simulink model "M12_MIMO_flexBitLoad_SVD"  (R2021a)
settings: Solver=FixedStepDiscrete  StartTime=0.0  StopTime=inf  RelTol=1e-3  EnableMultiTasking=on
undefined symbols (not defined in the file): B1, B2, BER, delay1, delay2, gcbh, L, magnitude, pl, pl1, pl2, rcfiltgaincompat, S, sigM1_g, sigM2_g, sigma, System, Tbit5_0, Tsk
libraries: simulink x8, dspstat3 x8, commfilt2 x4, commutil2 x2, commrandsrc3 x2, commdigbbndam3 x2, commsink2 x2, GeneralASKLib x2, NoiseLib_2021 x1, dspsrcs4 x1
settings Model: Creator=Praktikum  LastModifiedBy=st181028
settings SolverCC: AlgebraicLoopSolver=TrustRegion
settings DataIOCC: LimitDataPoints=on  SaveFormat=Array
settings OptimizationCC: ExpressionDepthLimit=2147483647  InitFltsAndDblsToZero=on  LifeSpan=inf
settings DebuggingCC: SaveWithDisabledLinksMsg=none  SaveWithParameterizedLinksMsg=none  SignalResolutionControl=TryResolveAllWithWarning  SolverPrmCheckMsg=warning  MultiTaskDSMMsg=warning  MultiTaskCondExecSysMsg=none  StateNameClashWarn=warning  StrictBusMsg=ErrorOnBusTreatedAsVector  SFUnexpectedBacktrackingDiag=warning  SFNoUnconditionalDefaultTransitionDiag=warning  SFMachineParentedDataDiag=warning  ArithmeticOperatorsInVariantConditions=warning
settings HardwareCC: ProdBitPerPointer=32  ProdBitPerSizeT=32  ProdBitPerPtrDiffT=32  ProdLargestAtomicFloat=None  ProdIntDivRoundTo=Undefined  ProdEndianess=Unspecified  ProdWordSize=32  ProdHWDeviceType=32-bit Generic
settings ModelReferenceCC: PropagateSignalLabelsOutOfModel=off
settings SFSimCC: SimUseLocalCustomCode=off  SimParseCustomCode=off  CustomCodeUndefinedFunction=UseInterfaceOnly
settings RTWCC: RTWUseLocalCustomCode=off
settings CodeAppCC: StateflowObjectComments=on
settings GRTTargetCC: TargetFcnLib=ansi_tfl_tmw.mat  TargetLangStandard=C89/C90 (ANSI)  CombineOutputUpdateFcns=off  GRTInterface=on
settings ConfigComp: CovMetricSettings=dw  CovSaveCumulativeToWorkspaceVar=on  CovSaveSingleToWorkspaceVar=on  CovExternalEMLEnable=off  CovSFcnEnable=off

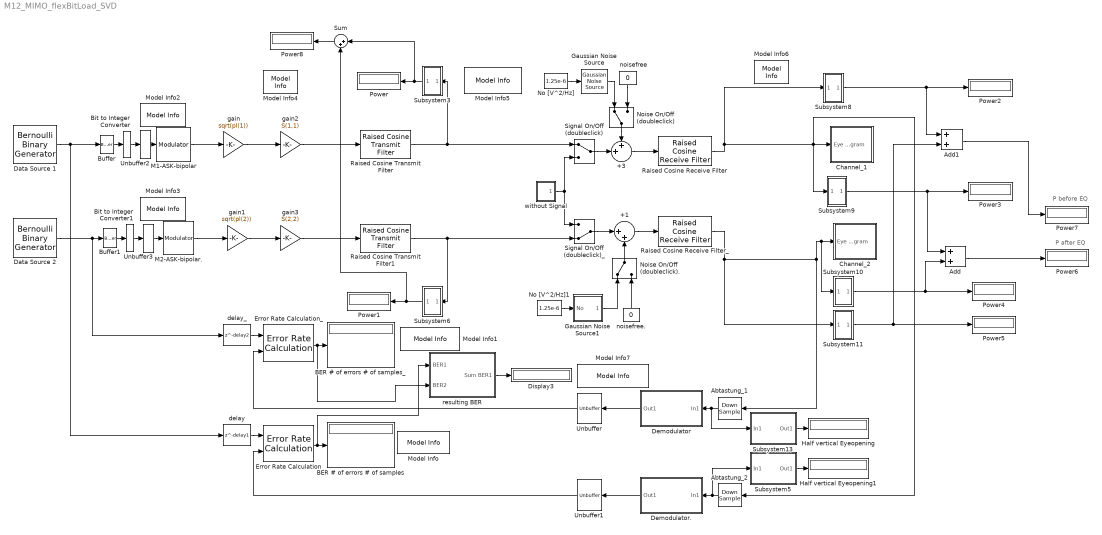
== system M12_MIMO_flexBitLoad_SVD ==
  note: P after EQ
  note: P before EQ
   Power{,1..8} (9 alike) : Display
  +1 : Sum  Inputs=|++  SampleTime=Tbit5_0/16
  +3 : Sum  Inputs=++|  SampleTime=Tbit5_0/16
  Abtastung_1 : DownSample  N=16  RateOptions=Allow multirate processing
  Abtastung_2 : DownSample  N=16  RateOptions=Allow multirate processing
  Add : Sum
  Add1 : Sum
  BER # of errors # of samples : Display
      settings: Format=short_e  Decimation=2
  BER # of errors # of samples_ : Display
      settings: Format=short_e  Decimation=2
  Bit to Integer Converter : commutil2/Bit to Integer Converter  nbits=B1  bitOrder=MSB first  signedOutputValues=Unsigned  outDtype=Inherit via internal rule  outDtypeSigned=Inherit via internal rule
  Bit to Integer Converter1 : commutil2/Bit to Integer Converter  nbits=B2  bitOrder=MSB first  signedOutputValues=Unsigned  outDtype=Inherit via internal rule  outDtypeSigned=Inherit via internal rule
  Buffer : Buffer  N=B1
  Buffer1 : Buffer  N=B2
  Channel_1 : Subsystem
  Channel_2 : Subsystem
  Data Source 1 : commrandsrc3/Bernoulli Binary Generator  ProbabilityOfZero=0.5  SeedSource=Parameter  Seed=61  SampleTime=Tbit5_0/B1  SamplesPerFrame=1  OutputDataType=double  SimulateUsing=Interpreted execution
  Data Source 2 : commrandsrc3/Bernoulli Binary Generator  ProbabilityOfZero=0.5  SeedSource=Parameter  Seed=51  SampleTime=Tbit5_0/B2  SamplesPerFrame=1  OutputDataType=double  SimulateUsing=Interpreted execution
  Demodulator : Subsystem  AncestorBlock=GeneralASKLib/Demodulator
      mask Display:
      | plot(0,0,100,100,[20+1.5*[[0:.8:10] [10:1.6:20] [20:.8:30]] 65 65 65 65+10*[0 1 1 2 2 3]],[85+10*[sin([0:.8:10]*pi*2/5) sin([10:1.6:20]*pi/5) sin([20:.8:30]*pi*2/5)] 85 99 75 85+8*[1 1 -1 -1 1 1]]);
      | disp('\nGeneral\nASK-Demodulator')
  Demodulator. : Subsystem  AncestorBlock=GeneralASKLib/Demodulator
      mask Display:
      | plot(0,0,100,100,[20+1.5*[[0:.8:10] [10:1.6:20] [20:.8:30]] 65 65 65 65+10*[0 1 1 2 2 3]],[85+10*[sin([0:.8:10]*pi*2/5) sin([10:1.6:20]*pi/5) sin([20:.8:30]*pi*2/5)] 85 99 75 85+8*[1 1 -1 -1 1 1]]);
      | disp('\nGeneral\nASK-Demodulator')
  Display3 : Display
      settings: Format=short_e
  Error Rate Calculation : commsink2/Error Rate Calculation  N=0  st_delay=100  cp_mode=Entire frame  subframe=1  PMode=Port  WsName=ErrorVec  RsMode2=off  stop=off  numErr=100  maxBits=1e6
  Error Rate Calculation_ : commsink2/Error Rate Calculation  N=0  st_delay=100  cp_mode=Entire frame  subframe=1  PMode=Port  WsName=ErrorVec  RsMode2=off  stop=off  numErr=100  maxBits=1e6
  Gaussian Noise Source : NoiseLib_2021/Gaussian Noise Source  SystemSampleTime=-1  VariantActivationTime=update diagram  Latency=0  AutoFrameSizeCalculation=off
  Gaussian Noise Source1 : Subsystem  AncestorBlock=NoiseLib_2021/Gaussian Noise Source
      mask Display:
      | plot(0,0,100,100,[95 5 10 10 10 (100-15)*[0:1/30:1]+10],[75 75 75 70 95 70    58 76 77 63 86 86 74 78 76 73 82 69 96 73 76 85 75 74 66 77 61 82 91 68    83 87 59 60 80 71]);
      | disp('\n\nGaussian')
      | port_label('input',1,'No')
      | port_label('output',1,'noise')
  Half vertical Eyeopening : Display
  Half vertical Eyeopening1 : Display
  M1-ASK-bipolar : GeneralASKLib/Modulator  SystemSampleTime=-1  VariantActivationTime=update diagram  Latency=0  AutoFrameSizeCalculation=off
      link override General ASK Modulator Baseband: SigCon=[sigM1_g]
  M2-ASK-bipolar. : GeneralASKLib/Modulator  SystemSampleTime=-1  VariantActivationTime=update diagram  Latency=0  AutoFrameSizeCalculation=off
      link override General ASK Modulator Baseband: SigCon=[sigM2_g]
  Model Info : simulink/Model-Wide Utilities/Model Info  Frame=off  DisplayStringWithTags=Channel_1  HorizontalTextAlignment=Center  LeftAlignmentValue=0.5
  Model Info1 : simulink/Model-Wide Utilities/Model Info  Frame=off  DisplayStringWithTags=Channel_2  HorizontalTextAlignment=Center  LeftAlignmentValue=0.5
  Model Info2 : simulink/Model-Wide Utilities/Model Info  Frame=off  DisplayStringWithTags=Channel1  HorizontalTextAlignment=Center  LeftAlignmentValue=0.5
  Model Info3 : simulink/Model-Wide Utilities/Model Info  Frame=off  DisplayStringWithTags=Channel2  HorizontalTextAlignment=Center  LeftAlignmentValue=0.5
  Model Info4 : simulink/Model-Wide Utilities/Model Info  Frame=off  DisplayStringWithTags=pre  HorizontalTextAlignment=Center  LeftAlignmentValue=0.5
  Model Info5 : simulink/Model-Wide Utilities/Model Info  Frame=off  DisplayStringWithTags=H  HorizontalTextAlignment=Center  LeftAlignmentValue=0.5
  Model Info6 : simulink/Model-Wide Utilities/Model Info  Frame=off  DisplayStringWithTags=pst  HorizontalTextAlignment=Center  LeftAlignmentValue=0.5
  Model Info7 : simulink/Model-Wide Utilities/Model Info  Frame=off  DisplayStringWithTags=System-BER  HorizontalTextAlignment=Center  LeftAlignmentValue=0.5
  No [V^2/Hz] : Constant  Value=1.25e-6
  No [V^2/Hz]1 : Constant  Value=1.25e-6
  Noise On/Off (doubleclick) : ManualSwitch
  Noise On/Off (doubleclick). : ManualSwitch
  Raised Cosine Receive Filter : commfilt2/Raised Cosine Receive Filter  filtType=Square root  R=0.5  filtSpan=2*(4)  N=16  downFactor=1  downOffset=0  filterGain=(0.25)*rcfiltgaincompat(gcbh)  RateOptions=Allow multirate processing  framing=Mute  checkCoeff=off  variableName=rcRxFilt  currentFiltSpan=2*(4)  D=4  inputOffset=0  sampMode=Mute  saveAsFlag=0  rateMode=Downsampling  checkGain=User-specified  launchFVT=off  roundingMode=Floor  overflowMode=off  coeffDataTypeStr=Inherit: Same word length as input  coeffMin=[]  coeffMax=[]  coeffLastDataTypeStr=Inherit: Same word length as input  accumDataTypeStr=Inherit: Same as product output  accumLastDataTypeStr=Inherit: Same as product output  outputDataTypeStr=Inherit: Same as accumulator  outputMin=[]  outputMax=[]  outputLastDataTypeStr=Inherit: Same as accumulator
  Raised Cosine Receive Filter_ : commfilt2/Raised Cosine Receive Filter  filtType=Square root  R=0.5  filtSpan=2*(4)  N=16  downFactor=1  downOffset=0  filterGain=(0.25)*rcfiltgaincompat(gcbh)  RateOptions=Allow multirate processing  framing=Mute  checkCoeff=off  variableName=rcRxFilt1  currentFiltSpan=2*(4)  D=4  inputOffset=0  sampMode=Mute  saveAsFlag=0  rateMode=Downsampling  checkGain=User-specified  launchFVT=off  roundingMode=Floor  overflowMode=off  coeffDataTypeStr=Inherit: Same word length as input  coeffMin=[]  coeffMax=[]  coeffLastDataTypeStr=Inherit: Same word length as input  accumDataTypeStr=Inherit: Same as product output  accumLastDataTypeStr=Inherit: Same as product output  outputDataTypeStr=Inherit: Same as accumulator  outputMin=[]  outputMax=[]  outputLastDataTypeStr=Inherit: Same as accumulator
  Raised Cosine Transmit Filter : commfilt2/Raised Cosine Transmit Filter  filtType=Square root  R=0.5  filtSpan=2*(4)  N=16  filterGain=(4/sqrt(2))*rcfiltgaincompat(gcbh)  RateOptions=Allow multirate processing  framing=Mute  checkCoeff=off  variableName=rcTxFilt  checkGain=User-specified  sampMode=Mute  saveAsFlag=0  currentFiltSpan=2*(4)  D=4  launchFVT=off  roundingMode=Floor  overflowMode=off  coeffDataTypeStr=Inherit: Same word length as input  coeffMin=[]  coeffMax=[]  coeffLastDataTypeStr=Inherit: Same word length as input  outputDataTypeStr=Inherit: Same as accumulator  outputMin=[]  outputMax=[]  outputLastDataTypeStr=Inherit: Same as accumulator
  Raised Cosine Transmit Filter1 : commfilt2/Raised Cosine Transmit Filter  filtType=Square root  R=0.5  filtSpan=2*(4)  N=16  filterGain=(4/sqrt(2))*rcfiltgaincompat(gcbh)  RateOptions=Allow multirate processing  framing=Mute  checkCoeff=off  variableName=rcTxFilt1  checkGain=User-specified  sampMode=Mute  saveAsFlag=0  currentFiltSpan=2*(4)  D=4  launchFVT=off  roundingMode=Floor  overflowMode=off  coeffDataTypeStr=Inherit: Same word length as input  coeffMin=[]  coeffMax=[]  coeffLastDataTypeStr=Inherit: Same word length as input  outputDataTypeStr=Inherit: Same as accumulator  outputMin=[]  outputMax=[]  outputLastDataTypeStr=Inherit: Same as accumulator
  Signal On/Off (doubleclick) : ManualSwitch
  Signal On/Off (doubleclick)_ : ManualSwitch  CurrentSetting=0
  Subsystem10 : Subsystem
      mask Display: disp('Power\n Measurement')
  Subsystem11 : Subsystem
      mask Display: disp('Power\n Measurement')
  Subsystem13 : Subsystem
      mask Display:
      | image('eye.bmp','center')
      | disp('\n\n\nEye Opening')
  Subsystem3 : Subsystem
      mask Display: disp('Power\n Measurement')
  Subsystem5 : Subsystem
      mask Display:
      | image('eye.bmp','center')
      | disp('\n\n\nEye Opening')
  Subsystem6 : Subsystem
      mask Display: disp('Power\n Measurement')
  Subsystem8 : Subsystem
      mask Display: disp('Power\n Measurement')
  Subsystem9 : Subsystem
      mask Display: disp('Power\n Measurement')
  Sum : Sum  Inputs=|++
  Unbuffer{,1..3} (4 alike) : Unbuffer
  delay : Delay  DelayLength=delay1  InitialCondition=0  InputProcessing=Columns as channels (frame based)
  delay_ : Delay  DelayLength=delay2  InitialCondition=0  InputProcessing=Columns as channels (frame based)
  gain : Gain  Gain=sqrt(pl(1))
  gain1 : Gain  Gain=sqrt(pl(2))
  gain2 : Gain  Gain=S(1,1)
  gain3 : Gain  Gain=S(2,2)
  noisefree : Constant  Value=0
  noisefree. : Constant  Value=0
  resulting BER : Subsystem
  without Signal : Subsystem
      mask Display: disp('0')
  wires:
  +3/1 -> Raised Cosine Receive Filter/1
  Signal On/Off (doubleclick)/1 -> +3/2
  Error Rate Calculation_/1 -> resulting BER/2(BER2), BER # of errors # of samples_/1
  delay_/1 -> Error Rate Calculation_/1
  Raised Cosine Transmit Filter/1 -> Signal On/Off (doubleclick)/1, Subsystem3/1(In1)
  without Signal/1(Out1) -> Signal On/Off (doubleclick)_/1, Signal On/Off (doubleclick)/2
  Raised Cosine Transmit Filter1/1 -> Signal On/Off (doubleclick)_/2, Subsystem6/1(In1)
  Error Rate Calculation/1 -> resulting BER/1(BER1), BER # of errors # of samples/1
  delay/1 -> Error Rate Calculation/1
  Raised Cosine Receive Filter_/1 -> Subsystem10/1(In1), Channel_2/1(Eye Diagram), Abtastung_1/1, Subsystem11/1(In1)
  Raised Cosine Receive Filter/1 -> Subsystem9/1(In1), Channel_1/1(Eye Diagram), Abtastung_2/1, Subsystem8/1(In1)
  Noise On/Off (doubleclick)/1 -> +3/1
  Abtastung_2/1 -> Subsystem5/1(In1), Demodulator./1(In1)
  Abtastung_1/1 -> Demodulator/1(In1), Subsystem13/1(In1)
  noisefree/1 -> Noise On/Off (doubleclick)/2
  No [V^2/Hz]/1 -> Gaussian Noise Source/1
  Gaussian Noise Source/1 -> Noise On/Off (doubleclick)/1
  Subsystem8/1(Out1) -> Add1/1, " Power2"/1
  Subsystem9/1(Out1) -> Add/1, " Power3"/1
  Subsystem10/1(Out1) -> Add/2, " Power4"/1
  Subsystem11/1(Out1) -> Add1/2, " Power5"/1
  Subsystem13/1(Out1) -> Half vertical Eyeopening/1
  Subsystem5/1(Out1) -> Half vertical Eyeopening1/1
  Subsystem3/1(Out1) -> Sum/1, " Power"/1
  Subsystem6/1(Out1) -> Sum/2, " Power1"/1
  +1/1 -> Raised Cosine Receive Filter_/1
  Signal On/Off (doubleclick)_/1 -> +1/1
  Noise On/Off (doubleclick)./1 -> +1/2
  noisefree./1 -> Noise On/Off (doubleclick)./2
  No [V^2/Hz]1/1 -> Gaussian Noise Source1/1(No)
  Gaussian Noise Source1/1(Noise) -> Noise On/Off (doubleclick)./1
  Unbuffer2/1 -> M1-ASK-bipolar/1
  Buffer/1 -> Bit to Integer Converter/1
  Bit to Integer Converter/1 -> Unbuffer2/1
  Unbuffer3/1 -> M2-ASK-bipolar./1
  Buffer1/1 -> Bit to Integer Converter1/1
  Bit to Integer Converter1/1 -> Unbuffer3/1
  resulting BER/1(Sum BER1) -> Display3/1
  Demodulator/1(Out1) -> Unbuffer/1
  Demodulator./1(Out1) -> Unbuffer1/1
  Unbuffer1/1 -> Error Rate Calculation/2
  Unbuffer/1 -> Error Rate Calculation_/2
  Add/1 -> " Power6"/1
  Add1/1 -> " Power7"/1
  Sum/1 -> " Power8"/1
  M1-ASK-bipolar/1 -> gain/1
  M2-ASK-bipolar./1 -> gain1/1
  Data Source 1/1 -> delay/1, Buffer/1
  Data Source 2/1 -> delay_/1, Buffer1/1
  gain/1 -> gain2/1
  gain2/1 -> Raised Cosine Transmit Filter/1
  gain1/1 -> gain3/1
  gain3/1 -> Raised Cosine Transmit Filter1/1

== system M12_MIMO_flexBitLoad_SVD/Channel_1 ==
  Eye Diagram : Inport
  Discrete-Time Eye Diagram Scope : EyeDiagram  Tag=EyeDiagram
  Realteil : ComplexToRealImag  Output=Real
  wires:
  Eye Diagram/1 -> Realteil/1
  Realteil/1 -> Discrete-Time Eye Diagram Scope/1

== system M12_MIMO_flexBitLoad_SVD/Channel_2 ==
  Eye Diagram : Inport
  Discrete-Time Eye Diagram Scope : EyeDiagram  Tag=EyeDiagram
  Realteil : ComplexToRealImag  Output=Real
  wires:
  Eye Diagram/1 -> Realteil/1
  Realteil/1 -> Discrete-Time Eye Diagram Scope/1

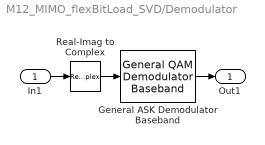
== system M12_MIMO_flexBitLoad_SVD/Demodulator ==
  In1 : Inport
  General ASK Demodulator Baseband : commdigbbndam3/General QAM Demodulator Baseband  SigCon=sigma(2)*sqrt(1/L)*sqrt(pl2)*sigM2_g  OutType=Bit  DecType=Hard decision  VarSource=Dialog  Variance=1  outDtypeBit=Inherit via internal rule  outDtype=Inherit via internal rule  roundingMode=Floor  overflowMode=Wrap  OvFlMode=off  OvFlModeLastStrValue=off  sigConstWordLen=16  sigConstDataTypeStr=Inherit: Same word length as input  sigConstLastDataTypeStr=Inherit: Same word length as input  accum1WordLen=32  accum1FracLen=30  prodInWordLen=32  prodInFracLen=30  prodInDataTypeStr=Inherit: Same as accumulator 1  prodInLastDataTypeStr=Inherit: Same as accumulator 1  prodOutWordLen=32  prodOutFracLen=30  accum2WordLen=32  accum2FracLen=30  accum3WordLen=32  accum3FracLen=30  nsiWordLen=32  nsiFracLen=30  nsiDataTypeStr=Inherit: Same as accumulator 3  nsiLastDataTypeStr=Inherit: Same as accumulator 3  invn0WordLen=16  invn0FracLen=8  invn0DataTypeStr=Inherit: Same word length as input  invn0LastDataTypeStr=Inherit: Same word length as input  outputWordLen=32  outputFracLen=30
      settings: SourceProductBaseCode=CM
  Real-Imag to Complex : RealImagToComplex  Input=Real
  Out1 : Outport
  wires:
  Real-Imag to Complex/1 -> General ASK Demodulator Baseband/1
  General ASK Demodulator Baseband/1 -> Out1/1
  In1/1 -> Real-Imag to Complex/1

== system M12_MIMO_flexBitLoad_SVD/Demodulator. ==
  In1 : Inport
  General ASK Demodulator Baseband : commdigbbndam3/General QAM Demodulator Baseband  SigCon=sigma(1)*sqrt(1/L)*sqrt(pl1)*sigM1_g  OutType=Bit  DecType=Hard decision  VarSource=Dialog  Variance=1  outDtypeBit=Inherit via internal rule  outDtype=Inherit via internal rule  roundingMode=Floor  overflowMode=Wrap  OvFlMode=off  OvFlModeLastStrValue=off  sigConstWordLen=16  sigConstDataTypeStr=Inherit: Same word length as input  sigConstLastDataTypeStr=Inherit: Same word length as input  accum1WordLen=32  accum1FracLen=30  prodInWordLen=32  prodInFracLen=30  prodInDataTypeStr=Inherit: Same as accumulator 1  prodInLastDataTypeStr=Inherit: Same as accumulator 1  prodOutWordLen=32  prodOutFracLen=30  accum2WordLen=32  accum2FracLen=30  accum3WordLen=32  accum3FracLen=30  nsiWordLen=32  nsiFracLen=30  nsiDataTypeStr=Inherit: Same as accumulator 3  nsiLastDataTypeStr=Inherit: Same as accumulator 3  invn0WordLen=16  invn0FracLen=8  invn0DataTypeStr=Inherit: Same word length as input  invn0LastDataTypeStr=Inherit: Same word length as input  outputWordLen=32  outputFracLen=30
      settings: SourceProductBaseCode=CM
  Real-Imag to Complex : RealImagToComplex  Input=Real
  Out1 : Outport
  wires:
  Real-Imag to Complex/1 -> General ASK Demodulator Baseband/1
  General ASK Demodulator Baseband/1 -> Out1/1
  In1/1 -> Real-Imag to Complex/1

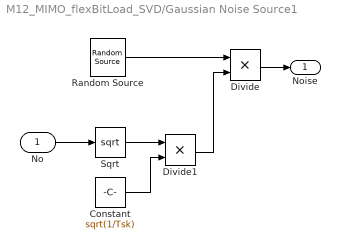
== system M12_MIMO_flexBitLoad_SVD/Gaussian Noise Source1 ==
  No : Inport
  Constant : Constant  Value=sqrt(1/Tsk)
  Divide : Product  Inputs=**
  Divide1 : Product  Inputs=**
  Random Source : dspsrcs4/Random Source  SrcType=Gaussian  NormMethod=Ziggurat  CltLength=12  MinVal=0  MaxVal=1  MeanVal=0  VarVal=1  RepMode=Specify seed  rawSeed=51  IsInherit=off  SampMode=Discrete  SampTime=Tsk  SampFrame=1  DataType=Double  OutComplex=Real  OutputFrames=off
  Sqrt : Sqrt  SaturateOnIntegerOverflow=on
  Noise : Outport
  wires:
  No/1 -> Sqrt/1
  Sqrt/1 -> Divide1/1
  Constant/1 -> Divide1/2
  Divide1/1 -> Divide/2
  Divide/1 -> Noise/1
  Random Source/1 -> Divide/1

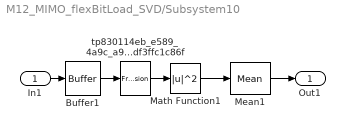
== system M12_MIMO_flexBitLoad_SVD/Subsystem10 ==
  In1 : Inport
  Buffer1 : Buffer  N=10*1024  OutputFrames=off
  Math Function1 : Math  Operator=magnitude^2  SignedPower=on  SaturateOnIntegerOverflow=on
  Mean1 : dspstat3/Mean  run=off  InputProcessing=Columns as channels (frame based)  reset_popup=None  directionMode=Each column  dimension=1  roiEnable=off  roiType=Rectangles  roiPortion=Entire ROI  roiOutput=Individual statistics for each ROI  roiFlag=off  roundingMode=Floor  overflowMode=off  outputDataTypeStr=Inherit: Same as accumulator  outputMin=[]  outputMax=[]  outputLastDataTypeStr=Inherit: Same as accumulator
  tp830114eb_e589_4a9c_a957_ddf3ffc1c86f : FrameConversion
  Out1 : Outport
  wires:
  Mean1/1 -> Out1/1
  In1/1 -> Buffer1/1
  Math Function1/1 -> Mean1/1
  Buffer1/1 -> tp830114eb_e589_4a9c_a957_ddf3ffc1c86f/1
  tp830114eb_e589_4a9c_a957_ddf3ffc1c86f/1 -> Math Function1/1

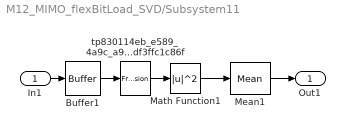
== system M12_MIMO_flexBitLoad_SVD/Subsystem11 ==
  In1 : Inport
  Buffer1 : Buffer  N=10*1024  OutputFrames=off
  Math Function1 : Math  Operator=magnitude^2  SignedPower=on  SaturateOnIntegerOverflow=on
  Mean1 : dspstat3/Mean  run=off  InputProcessing=Columns as channels (frame based)  reset_popup=None  directionMode=Each column  dimension=1  roiEnable=off  roiType=Rectangles  roiPortion=Entire ROI  roiOutput=Individual statistics for each ROI  roiFlag=off  roundingMode=Floor  overflowMode=off  outputDataTypeStr=Inherit: Same as accumulator  outputMin=[]  outputMax=[]  outputLastDataTypeStr=Inherit: Same as accumulator
  tp830114eb_e589_4a9c_a957_ddf3ffc1c86f : FrameConversion
  Out1 : Outport
  wires:
  Mean1/1 -> Out1/1
  In1/1 -> Buffer1/1
  Math Function1/1 -> Mean1/1
  Buffer1/1 -> tp830114eb_e589_4a9c_a957_ddf3ffc1c86f/1
  tp830114eb_e589_4a9c_a957_ddf3ffc1c86f/1 -> Math Function1/1

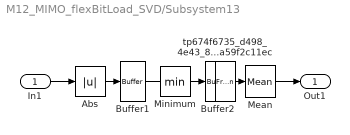
== system M12_MIMO_flexBitLoad_SVD/Subsystem13 ==
  In1 : Inport
  Abs : Abs
  Buffer1 : Buffer  N=20  V=4  OutputFrames=off
  Buffer2 : Buffer  N=200  V=4
  Mean : dspstat3/Mean  run=off  InputProcessing=Columns as channels (frame based)  reset_popup=None  directionMode=Each column  dimension=1  roiEnable=off  roiType=Rectangles  roiPortion=Entire ROI  roiOutput=Individual statistics for each ROI  roiFlag=off  roundingMode=Floor  overflowMode=off  outputDataTypeStr=Inherit: Same as accumulator  outputMin=[]  outputMax=[]  outputLastDataTypeStr=Inherit: Same as accumulator
  Minimum : MinMax
  tp674f6735_d498_4e43_822c_fba59f2c11ec : FrameConversion
  Out1 : Outport
  wires:
  Abs/1 -> Buffer1/1
  Minimum/1 -> Buffer2/1
  Buffer2/1 -> Mean/1
  In1/1 -> Abs/1
  Mean/1 -> Out1/1
  Buffer1/1 -> tp674f6735_d498_4e43_822c_fba59f2c11ec/1
  tp674f6735_d498_4e43_822c_fba59f2c11ec/1 -> Minimum/1

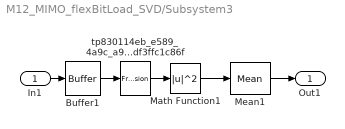
== system M12_MIMO_flexBitLoad_SVD/Subsystem3 ==
  In1 : Inport
  Buffer1 : Buffer  N=10*1024  OutputFrames=off
  Math Function1 : Math  Operator=magnitude^2  SignedPower=on  SaturateOnIntegerOverflow=on
  Mean1 : dspstat3/Mean  run=off  InputProcessing=Columns as channels (frame based)  reset_popup=None  directionMode=Each column  dimension=1  roiEnable=off  roiType=Rectangles  roiPortion=Entire ROI  roiOutput=Individual statistics for each ROI  roiFlag=off  roundingMode=Floor  overflowMode=off  outputDataTypeStr=Inherit: Same as accumulator  outputMin=[]  outputMax=[]  outputLastDataTypeStr=Inherit: Same as accumulator
  tp830114eb_e589_4a9c_a957_ddf3ffc1c86f : FrameConversion
  Out1 : Outport
  wires:
  Mean1/1 -> Out1/1
  In1/1 -> Buffer1/1
  Math Function1/1 -> Mean1/1
  Buffer1/1 -> tp830114eb_e589_4a9c_a957_ddf3ffc1c86f/1
  tp830114eb_e589_4a9c_a957_ddf3ffc1c86f/1 -> Math Function1/1

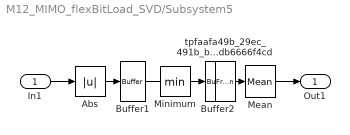
== system M12_MIMO_flexBitLoad_SVD/Subsystem5 ==
  In1 : Inport
  Abs : Abs
  Buffer1 : Buffer  N=20  V=4  OutputFrames=off
  Buffer2 : Buffer  N=200  V=4
  Mean : dspstat3/Mean  run=off  InputProcessing=Columns as channels (frame based)  reset_popup=None  directionMode=Each column  dimension=1  roiEnable=off  roiType=Rectangles  roiPortion=Entire ROI  roiOutput=Individual statistics for each ROI  roiFlag=off  roundingMode=Floor  overflowMode=off  outputDataTypeStr=Inherit: Same as accumulator  outputMin=[]  outputMax=[]  outputLastDataTypeStr=Inherit: Same as accumulator
  Minimum : MinMax
  tpfaafa49b_29ec_491b_b872_1ddb6666f4cd : FrameConversion
  Out1 : Outport
  wires:
  Abs/1 -> Buffer1/1
  Minimum/1 -> Buffer2/1
  Buffer2/1 -> Mean/1
  In1/1 -> Abs/1
  Mean/1 -> Out1/1
  Buffer1/1 -> tpfaafa49b_29ec_491b_b872_1ddb6666f4cd/1
  tpfaafa49b_29ec_491b_b872_1ddb6666f4cd/1 -> Minimum/1

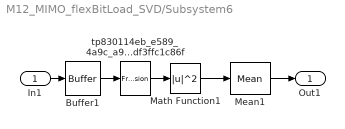
== system M12_MIMO_flexBitLoad_SVD/Subsystem6 ==
  In1 : Inport
  Buffer1 : Buffer  N=10*1024  OutputFrames=off
  Math Function1 : Math  Operator=magnitude^2  SignedPower=on  SaturateOnIntegerOverflow=on
  Mean1 : dspstat3/Mean  run=off  InputProcessing=Columns as channels (frame based)  reset_popup=None  directionMode=Each column  dimension=1  roiEnable=off  roiType=Rectangles  roiPortion=Entire ROI  roiOutput=Individual statistics for each ROI  roiFlag=off  roundingMode=Floor  overflowMode=off  outputDataTypeStr=Inherit: Same as accumulator  outputMin=[]  outputMax=[]  outputLastDataTypeStr=Inherit: Same as accumulator
  tp830114eb_e589_4a9c_a957_ddf3ffc1c86f : FrameConversion
  Out1 : Outport
  wires:
  Mean1/1 -> Out1/1
  In1/1 -> Buffer1/1
  Math Function1/1 -> Mean1/1
  Buffer1/1 -> tp830114eb_e589_4a9c_a957_ddf3ffc1c86f/1
  tp830114eb_e589_4a9c_a957_ddf3ffc1c86f/1 -> Math Function1/1

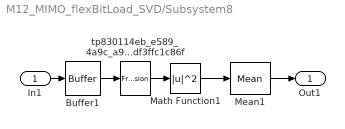
== system M12_MIMO_flexBitLoad_SVD/Subsystem8 ==
  In1 : Inport
  Buffer1 : Buffer  N=10*1024  OutputFrames=off
  Math Function1 : Math  Operator=magnitude^2  SignedPower=on  SaturateOnIntegerOverflow=on
  Mean1 : dspstat3/Mean  run=off  InputProcessing=Columns as channels (frame based)  reset_popup=None  directionMode=Each column  dimension=1  roiEnable=off  roiType=Rectangles  roiPortion=Entire ROI  roiOutput=Individual statistics for each ROI  roiFlag=off  roundingMode=Floor  overflowMode=off  outputDataTypeStr=Inherit: Same as accumulator  outputMin=[]  outputMax=[]  outputLastDataTypeStr=Inherit: Same as accumulator
  tp830114eb_e589_4a9c_a957_ddf3ffc1c86f : FrameConversion
  Out1 : Outport
  wires:
  Mean1/1 -> Out1/1
  In1/1 -> Buffer1/1
  Math Function1/1 -> Mean1/1
  Buffer1/1 -> tp830114eb_e589_4a9c_a957_ddf3ffc1c86f/1
  tp830114eb_e589_4a9c_a957_ddf3ffc1c86f/1 -> Math Function1/1

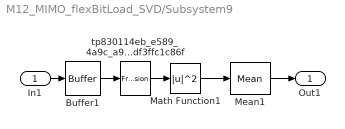
== system M12_MIMO_flexBitLoad_SVD/Subsystem9 ==
  In1 : Inport
  Buffer1 : Buffer  N=10*1024  OutputFrames=off
  Math Function1 : Math  Operator=magnitude^2  SignedPower=on  SaturateOnIntegerOverflow=on
  Mean1 : dspstat3/Mean  run=off  InputProcessing=Columns as channels (frame based)  reset_popup=None  directionMode=Each column  dimension=1  roiEnable=off  roiType=Rectangles  roiPortion=Entire ROI  roiOutput=Individual statistics for each ROI  roiFlag=off  roundingMode=Floor  overflowMode=off  outputDataTypeStr=Inherit: Same as accumulator  outputMin=[]  outputMax=[]  outputLastDataTypeStr=Inherit: Same as accumulator
  tp830114eb_e589_4a9c_a957_ddf3ffc1c86f : FrameConversion
  Out1 : Outport
  wires:
  Mean1/1 -> Out1/1
  In1/1 -> Buffer1/1
  Math Function1/1 -> Mean1/1
  Buffer1/1 -> tp830114eb_e589_4a9c_a957_ddf3ffc1c86f/1
  tp830114eb_e589_4a9c_a957_ddf3ffc1c86f/1 -> Math Function1/1

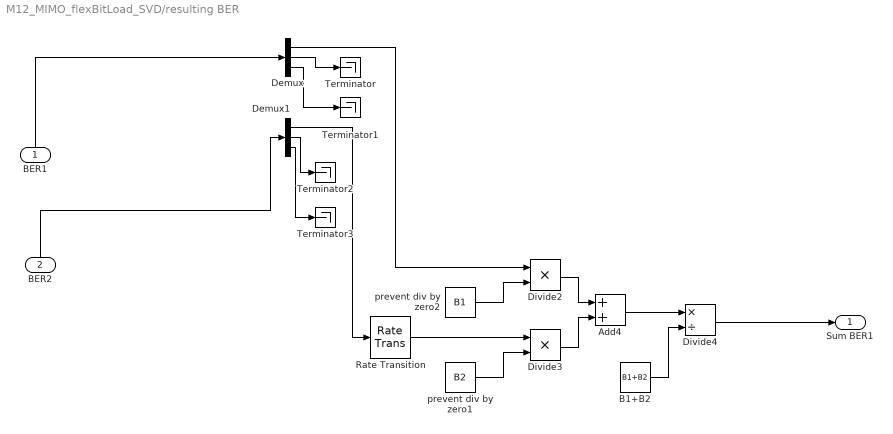
== system M12_MIMO_flexBitLoad_SVD/resulting BER ==
  BER1 : Inport
  BER2 : Inport  Port=2
  Add4 : Sum
  B1+B2 : Constant  Value=B1+B2
  Demux : Demux  Outputs=3
  Demux1 : Demux  Outputs=3
  Divide2 : Product  Inputs=**
  Divide3 : Product  Inputs=**
  Divide4 : Product  Inputs=*/
  Rate Transition : RateTransition  Deterministic=off
  Terminator{,1..3} (4 alike) : Terminator
  prevent div by zero1 : Constant  Value=B2
  prevent div by zero2 : Constant  Value=B1
  Sum BER1 : Outport
  wires:
  Demux1/3 -> Terminator3/1
  Demux1/2 -> Terminator2/1
  Demux/2 -> Terminator/1
  Demux/3 -> Terminator1/1
  Rate Transition/1 -> Divide3/1
  Divide4/1 -> Sum BER1/1
  B1+B2/1 -> Divide4/2
  Add4/1 -> Divide4/1
  Divide3/1 -> Add4/2
  Divide2/1 -> Add4/1
  prevent div by zero1/1 -> Divide3/2
  prevent div by zero2/1 -> Divide2/2
  BER1/1 -> Demux/1
  BER2/1 -> Demux1/1
  Demux1/1 -> Rate Transition/1
  Demux/1 -> Divide2/1

== system M12_MIMO_flexBitLoad_SVD/without Signal ==
  Konstante : Constant  Value=0  OutDataTypeStr=double
  Out1 : Outport
  wires:
  Konstante/1 -> Out1/1
